simulink model "Ini_SO3_model_MixedCZ"  (R2021a)
settings: Solver=ode4  StartTime=0.0  StopTime=1000  FixedStep=0.02  RelTol=1e-3
values from neighbouring files (symbols this model uses):
  alpha = 0.05    [Ini_SO3.m]    (also in Ini_SO3_MixedCZ.m = 0.3; coneNew.m = acos(cosalpha))
  beta = 0.05    [Ini_SO3.m]    (also in Ini_SO3_MixedCZ.m = 0.3)
  G = [1,0,0 ... (first row only)    [Ini_SO3.m]    (also in Ini_SO3_MixedCZ.m; Symmetric test.m = inv(J)*D*E*D')
  J0 = [60 0 -5 ... (first row only)    [Ini_SO3.m]    (also in Ini_SO3_MixedCZ.m)
  J1 = [60 0 -5 ... (first row only)    [Ini_SO3.m]    (also in Ini_SO3_MixedCZ.m)
  J2 = [60 0 -5 ... (first row only)    [Ini_SO3.m]    (also in Ini_SO3_MixedCZ.m)
  J3 = [60 0 -5 ... (first row only)    [Ini_SO3.m]    (also in Ini_SO3_MixedCZ.m)
  K = [0.5,5,25,0.5]'    [Ini_SO3_MixedCZ.m]
  K1 = [0.01,0,30,0.2]'    [Ini_SO3.m]    (also in Ini_SO3_MixedCZ.m = [0.01,0,30,0.1]')
  lambda = 0.05    [Ini_SO3.m]    (also in Ini_SO3_MixedCZ.m = 0.3; SO3toThetan.m = diag(lambda))
  Omega01 = [0.03;0.02;-0.03]    [Ini_SO3.m]    (also in Ini_SO3_MixedCZ.m = [0,0,0])
  Omega02 = [-0.02;0.02;-0.03]    [Ini_SO3.m]    (also in Ini_SO3_MixedCZ.m = [0,0,0])
  Omega03 = [0;0.03;0.04]    [Ini_SO3.m]    (also in Ini_SO3_MixedCZ.m = [0,0,0])
  Omega0d = [0;0;0]    [Ini_SO3.m]    (also in Ini_SO3_MixedCZ.m)
  R01 = SO3(deg2rad(-80), nd0)    [Ini_SO3.m]    (also in Ini_SO3_MixedCZ.m = SO3(2.387, [0.3145,0.9113,0.2658]'))
  R02 = SO3(deg2rad(40),[0;1;1]/norm([0;1;1]))    [Ini_SO3.m]    (also in Ini_SO3_MixedCZ.m = SO3(1.422, [0.1772,0.9751,-0.1329]'))
  R03 = SO3(deg2rad(-120), nd0)    [Ini_SO3.m]    (also in Ini_SO3_MixedCZ.m = SO3(2.007, [0.2997,0.9415,0.1543]'))
  Rd = SO3(-(2*pi-Angd),nd)    [Ini_SO3.m]    (also in Ini_SO3_MixedCZ.m = SO3(Angd,nd))
  Rd0 = SO3(-(2*pi-Angd0),nd0)    [Ini_SO3.m]    (also in Ini_SO3_MixedCZ.m = SO3(Angd0,nd0))
  X = zeros(4,4)    [Ini_SO3.m]    (also in Ini_SO3_MixedCZ.m; coneNew.m = R .* cos(A))
undefined symbols (not defined in the file or in its folder): deg, rad, s
libraries: aerolibconvert2 x8
settings Model: Creator=Zeyu  LastModifiedBy=泽禹

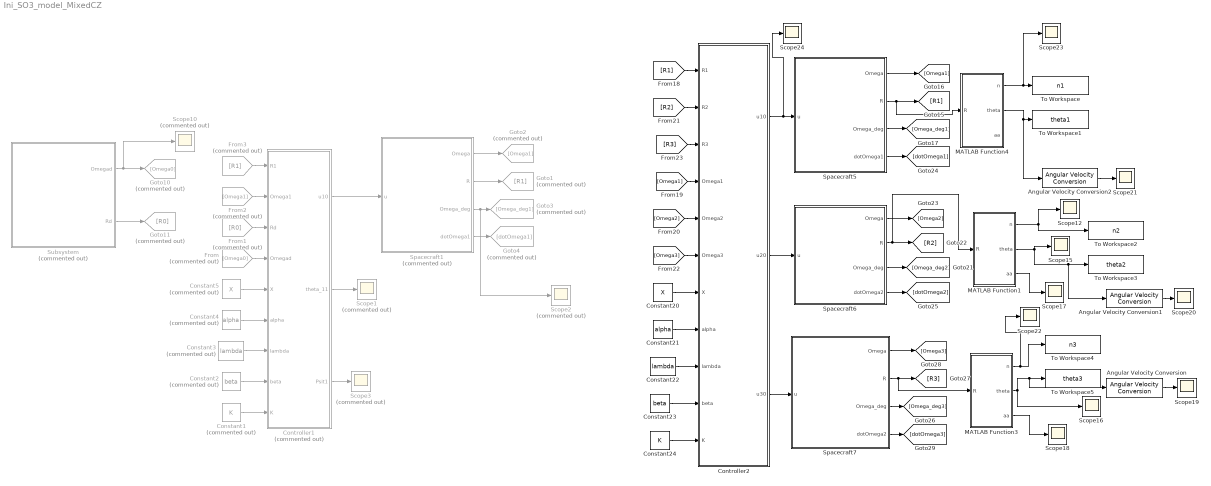
== system Ini_SO3_model_MixedCZ ==
  Angular Velocity Conversion : aerolibconvert2/Angular Velocity Conversion  IU=rad/s  OU=deg/s
  Angular Velocity Conversion1 : aerolibconvert2/Angular Velocity Conversion  IU=rad/s  OU=deg/s
  Angular Velocity Conversion2 : aerolibconvert2/Angular Velocity Conversion  IU=rad/s  OU=deg/s
  Constant1 : Constant  Commented=on  Value=K
  Constant2 : Constant  Commented=on  Value=beta
  Constant20 : Constant  Value=X
  Constant21 : Constant  Value=alpha
  Constant22 : Constant  Value=lambda
  Constant23 : Constant  Value=beta
  Constant24 : Constant  Value=K
  Constant3 : Constant  Commented=on  Value=lambda
  Constant4 : Constant  Commented=on  Value=alpha
  Constant5 : Constant  Commented=on  Value=X
  Controller1 : MATLAB Function  Commented=on  TreatAsAtomicUnit=on
  Controller2 : MATLAB Function  TreatAsAtomicUnit=on
  From : From  Commented=on  GotoTag=Omega0
  From1 : From  Commented=on  GotoTag=R0
  From2 : From  Commented=on  GotoTag=Omega1
  From3 : From  Commented=on  GotoTag=R1
  Goto1 : Goto  Commented=on  GotoTag=R1
  Goto10 : Goto  Commented=on  GotoTag=Omega0
  Goto11 : Goto  Commented=on  GotoTag=R0
  Goto2 : Goto  Commented=on  GotoTag=Omega1
  Goto3 : Goto  Commented=on  GotoTag=Omega_deg1
  Goto4 : Goto  Commented=on  GotoTag=dotOmega1
  MATLAB Function1 : MATLAB Function  TreatAsAtomicUnit=on
  MATLAB Function3 : MATLAB Function  TreatAsAtomicUnit=on
  MATLAB Function4 : MATLAB Function  TreatAsAtomicUnit=on
  Scope{1..3,10} (4 alike) : Scope  Commented=on
  Scope{12,15..24} (11 alike) : Scope
  Spacecraft1 : Subsystem  Commented=on
  Spacecraft5 : Subsystem
  Spacecraft6 : Subsystem
  Spacecraft7 : Subsystem
  Subsystem : Subsystem  Commented=on
  To Workspace : ToWorkspace  VariableName=n1  SampleTime=-1
  To Workspace1 : ToWorkspace  VariableName=theta1  SampleTime=-1
  To Workspace2 : ToWorkspace  VariableName=n2  SampleTime=-1
  To Workspace3 : ToWorkspace  VariableName=theta2  SampleTime=-1
  To Workspace4 : ToWorkspace  VariableName=n3  SampleTime=-1
  To Workspace5 : ToWorkspace  VariableName=theta3  SampleTime=-1
  wires:
  Spacecraft5/4(dotOmega1) -> [dotOmega1]
  Spacecraft5/3(Omega_deg) -> [Omega_deg1]
  Spacecraft6/3(Omega_deg) -> [Omega_deg2]
  Spacecraft6/1(Omega) -> [Omega2]
  Spacecraft6/4(dotOmega2) -> [dotOmega2]
  Spacecraft5/1(Omega) -> [Omega1]
  Spacecraft5/2(R) -> MATLAB Function4/1(R), [R1]
  Controller2/2(u20) -> Spacecraft6/1(u)
  Controller2/1(u10) -> Scope24/1, Spacecraft5/1(u)
  [R1] -> Controller2/1(R1)
  [Omega1] -> Controller2/4(Omega1)
  [Omega2] -> Controller2/5(Omega2)
  [R2] -> Controller2/2(R2)
  Constant20/1 -> Controller2/7(X)
  Constant21/1 -> Controller2/8(alpha)
  Constant22/1 -> Controller2/9(lambda)
  Constant23/1 -> Controller2/10(beta)
  Constant24/1 -> Controller2/11(K)
  Spacecraft7/3(Omega_deg) -> [Omega_deg3]
  Spacecraft7/4(dotOmega2) -> [dotOmega3]
  Controller2/3(u30) -> Spacecraft7/1(u)
  Spacecraft7/1(Omega) -> [Omega3]
  [Omega3] -> Controller2/6(Omega3)
  [R3] -> Controller2/3(R3)
  Spacecraft6/2(R) -> MATLAB Function1/1(R), [R2]
  Spacecraft7/2(R) -> MATLAB Function3/1(R), [R3]
  MATLAB Function4/1(n) -> Scope23/1, To Workspace/1
  MATLAB Function1/2(theta) -> Angular Velocity Conversion1/1, To Workspace3/1, Scope15/1
  MATLAB Function1/1(n) -> To Workspace2/1, Scope12/1
  MATLAB Function3/1(n) -> Scope22/1, To Workspace4/1
  MATLAB Function3/2(theta) -> Scope16/1, Angular Velocity Conversion/1, To Workspace5/1
  MATLAB Function1/3(aa) -> Scope17/1
  MATLAB Function3/3(aa) -> Scope18/1
  Angular Velocity Conversion/1 -> Scope19/1
  Angular Velocity Conversion1/1 -> Scope20/1
  Angular Velocity Conversion2/1 -> Scope21/1
  MATLAB Function4/2(theta) -> Angular Velocity Conversion2/1, To Workspace1/1
  Subsystem/2(Rd) -> Goto11/1
  Subsystem/1(Omegad) -> Scope10/1, Goto10/1
  Spacecraft1/2(R) -> Goto1/1
  Spacecraft1/3(Omega_deg) -> Scope2/1, Goto3/1
  Spacecraft1/1(Omega) -> Goto2/1
  Spacecraft1/4(dotOmega1) -> Goto4/1
  Controller1/1(u10) -> Spacecraft1/1(u)
  Constant1/1 -> Controller1/9(K)
  Controller1/2(theta_11) -> Scope1/1
  Constant2/1 -> Controller1/8(beta)
  Constant3/1 -> Controller1/7(lambda)
  Constant4/1 -> Controller1/6(alpha)
  Constant5/1 -> Controller1/5(X)
  From/1 -> Controller1/4(Omegad)
  From1/1 -> Controller1/3(Rd)
  From2/1 -> Controller1/2(Omega1)
  From3/1 -> Controller1/1(R1)
  Controller1/3(Psit1) -> Scope3/1

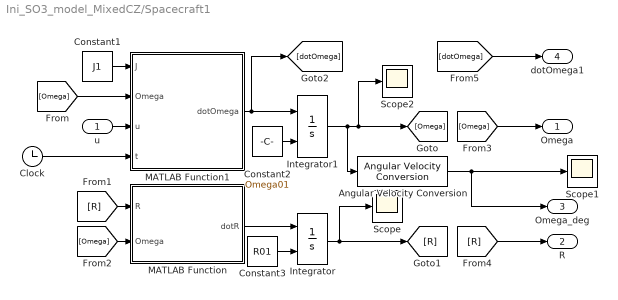
== system Ini_SO3_model_MixedCZ/Spacecraft1 ==
  u : Inport
  Angular Velocity Conversion : aerolibconvert2/Angular Velocity Conversion  IU=rad/s  OU=deg/s
  Clock : Clock
  Constant1 : Constant  Value=J1
  Constant2 : Constant  Value=Omega01
  Constant3 : Constant  Value=R01
  Integrator : Integrator  InitialConditionSource=external
  Integrator1 : Integrator  InitialConditionSource=external
  MATLAB Function : MATLAB Function  TreatAsAtomicUnit=on
  MATLAB Function1 : MATLAB Function  TreatAsAtomicUnit=on
  Scope : Scope
  Scope1 : Scope
  Scope2 : Scope
  Omega : Outport
  R : Outport  Port=2
  Omega_deg : Outport  Port=3
  dotOmega1 : Outport  Port=4
  wires:
  Constant3/1 -> Integrator/2
  Integrator/1 -> [R], Scope/1
  Constant1/1 -> MATLAB Function1/1(J)
  Integrator1/1 -> Scope2/1, [Omega], Angular Velocity Conversion/1
  MATLAB Function1/1(dotOmega) -> [dotOmega], Integrator1/1
  [Omega] -> MATLAB Function/2(Omega)
  MATLAB Function/1(dotR) -> Integrator/1
  Constant2/1 -> Integrator1/2
  [Omega] -> MATLAB Function1/2(Omega)
  [R] -> MATLAB Function/1(R)
  Angular Velocity Conversion/1 -> Omega_deg/1, Scope1/1
  u/1 -> MATLAB Function1/3(u)
  [Omega] -> Omega/1
  [R] -> R/1
  Clock/1 -> MATLAB Function1/4(t)
  [dotOmega] -> dotOmega1/1

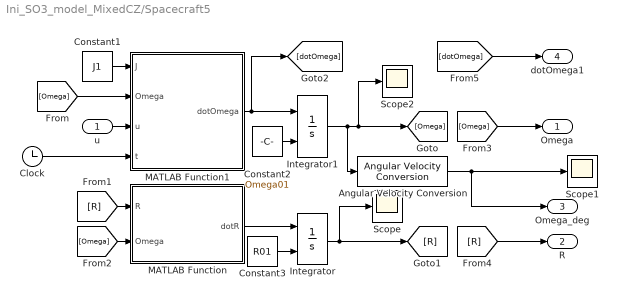
== system Ini_SO3_model_MixedCZ/Spacecraft5 ==
  u : Inport
  Angular Velocity Conversion : aerolibconvert2/Angular Velocity Conversion  IU=rad/s  OU=deg/s
  Clock : Clock
  Constant1 : Constant  Value=J1
  Constant2 : Constant  Value=Omega01
  Constant3 : Constant  Value=R01
  Integrator : Integrator  InitialConditionSource=external
  Integrator1 : Integrator  InitialConditionSource=external
  MATLAB Function : MATLAB Function  TreatAsAtomicUnit=on
  MATLAB Function1 : MATLAB Function  TreatAsAtomicUnit=on
  Scope : Scope
  Scope1 : Scope
  Scope2 : Scope
  Omega : Outport
  R : Outport  Port=2
  Omega_deg : Outport  Port=3
  dotOmega1 : Outport  Port=4
  wires:
  Constant3/1 -> Integrator/2
  Integrator/1 -> [R], Scope/1
  Constant1/1 -> MATLAB Function1/1(J)
  Integrator1/1 -> Scope2/1, [Omega], Angular Velocity Conversion/1
  MATLAB Function1/1(dotOmega) -> [dotOmega], Integrator1/1
  [Omega] -> MATLAB Function/2(Omega)
  MATLAB Function/1(dotR) -> Integrator/1
  Constant2/1 -> Integrator1/2
  [Omega] -> MATLAB Function1/2(Omega)
  [R] -> MATLAB Function/1(R)
  Angular Velocity Conversion/1 -> Omega_deg/1, Scope1/1
  u/1 -> MATLAB Function1/3(u)
  [Omega] -> Omega/1
  [R] -> R/1
  Clock/1 -> MATLAB Function1/4(t)
  [dotOmega] -> dotOmega1/1

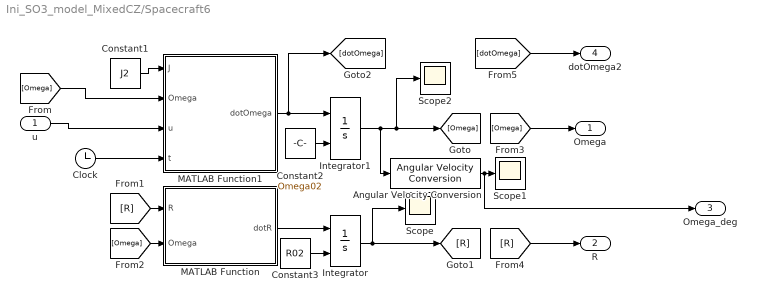
== system Ini_SO3_model_MixedCZ/Spacecraft6 ==
  u : Inport
  Angular Velocity Conversion : aerolibconvert2/Angular Velocity Conversion  IU=rad/s  OU=deg/s
  Clock : Clock
  Constant1 : Constant  Value=J2
  Constant2 : Constant  Value=Omega02
  Constant3 : Constant  Value=R02
  Integrator : Integrator  InitialConditionSource=external
  Integrator1 : Integrator  InitialConditionSource=external
  MATLAB Function : MATLAB Function  TreatAsAtomicUnit=on
  MATLAB Function1 : MATLAB Function  TreatAsAtomicUnit=on
  Scope : Scope
  Scope1 : Scope
  Scope2 : Scope
  Omega : Outport
  R : Outport  Port=2
  Omega_deg : Outport  Port=3
  dotOmega2 : Outport  Port=4
  wires:
  Constant3/1 -> Integrator/2
  Integrator/1 -> [R], Scope/1
  Constant1/1 -> MATLAB Function1/1(J)
  [Omega] -> MATLAB Function/2(Omega)
  MATLAB Function/1(dotR) -> Integrator/1
  Constant2/1 -> Integrator1/2
  [Omega] -> MATLAB Function1/2(Omega)
  [R] -> MATLAB Function/1(R)
  u/1 -> MATLAB Function1/3(u)
  [Omega] -> Omega/1
  [R] -> R/1
  Clock/1 -> MATLAB Function1/4(t)
  Angular Velocity Conversion/1 -> Omega_deg/1, Scope1/1
  Integrator1/1 -> Scope2/1, [Omega], Angular Velocity Conversion/1
  [dotOmega] -> dotOmega2/1
  MATLAB Function1/1(dotOmega) -> [dotOmega], Integrator1/1

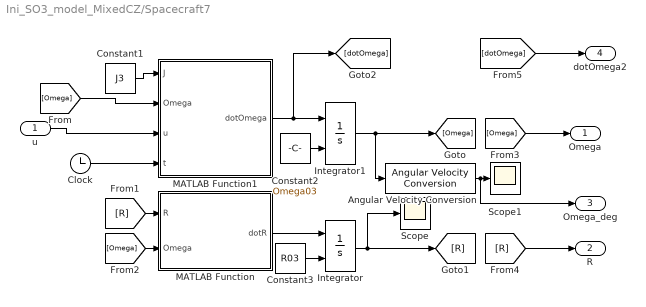
== system Ini_SO3_model_MixedCZ/Spacecraft7 ==
  u : Inport
  Angular Velocity Conversion : aerolibconvert2/Angular Velocity Conversion  IU=rad/s  OU=deg/s
  Clock : Clock
  Constant1 : Constant  Value=J3
  Constant2 : Constant  Value=Omega03
  Constant3 : Constant  Value=R03
  Integrator : Integrator  InitialConditionSource=external
  Integrator1 : Integrator  InitialConditionSource=external
  MATLAB Function : MATLAB Function  TreatAsAtomicUnit=on
  MATLAB Function1 : MATLAB Function  TreatAsAtomicUnit=on
  Scope : Scope
  Scope1 : Scope
  Omega : Outport
  R : Outport  Port=2
  Omega_deg : Outport  Port=3
  dotOmega2 : Outport  Port=4
  wires:
  Constant3/1 -> Integrator/2
  Integrator/1 -> [R], Scope/1
  Constant1/1 -> MATLAB Function1/1(J)
  Integrator1/1 -> [Omega], Angular Velocity Conversion/1
  [Omega] -> MATLAB Function/2(Omega)
  MATLAB Function/1(dotR) -> Integrator/1
  Constant2/1 -> Integrator1/2
  [Omega] -> MATLAB Function1/2(Omega)
  [R] -> MATLAB Function/1(R)
  u/1 -> MATLAB Function1/3(u)
  [Omega] -> Omega/1
  [R] -> R/1
  Clock/1 -> MATLAB Function1/4(t)
  Angular Velocity Conversion/1 -> Omega_deg/1, Scope1/1
  MATLAB Function1/1(dotOmega) -> [dotOmega], Integrator1/1
  [dotOmega] -> dotOmega2/1

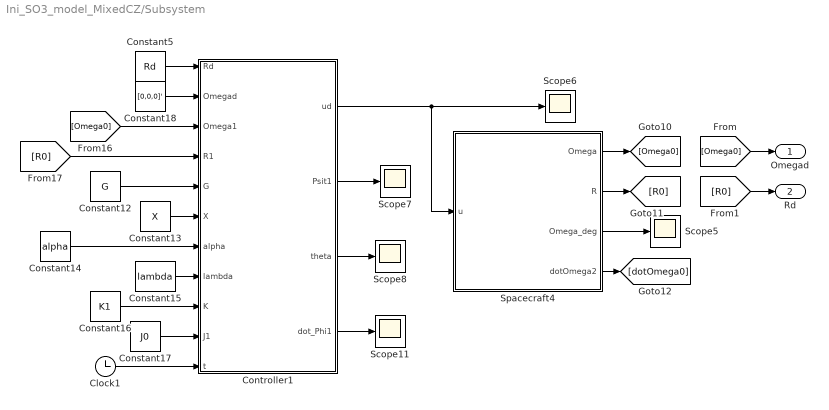
== system Ini_SO3_model_MixedCZ/Subsystem ==
  Clock1 : Clock
  Constant12 : Constant  Value=G
  Constant13 : Constant  Value=X
  Constant14 : Constant  Value=alpha
  Constant15 : Constant  Value=lambda
  Constant16 : Constant  Value=K1
  Constant17 : Constant  Value=J0
  Constant18 : Constant  Value=[0,0,0]'
  Constant5 : Constant  Value=Rd
  Controller1 : MATLAB Function  TreatAsAtomicUnit=on
  Scope{5..8,11} (5 alike) : Scope
  Spacecraft4 : Subsystem
  Omegad : Outport
  Rd : Outport  Port=2
  wires:
  Spacecraft4/4(dotOmega2) -> [dotOmega0]
  [R0] -> Controller1/4(R1)
  Controller1/1(ud) -> Scope6/1, Spacecraft4/1(u)
  Constant16/1 -> Controller1/9(K)
  Constant12/1 -> Controller1/5(G)
  Constant18/1 -> Controller1/2(Omegad)
  Constant17/1 -> Controller1/10(J1)
  Constant5/1 -> Controller1/1(Rd)
  Constant14/1 -> Controller1/7(alpha)
  Constant15/1 -> Controller1/8(lambda)
  Constant13/1 -> Controller1/6(X)
  Clock1/1 -> Controller1/11(t)
  [Omega0] -> Controller1/3(Omega1)
  Controller1/4(dot_Phi1) -> Scope11/1
  Controller1/3(theta) -> Scope8/1
  Spacecraft4/3(Omega_deg) -> Scope5/1
  Controller1/2(Psit1) -> Scope7/1
  Spacecraft4/2(R) -> [R0]
  Spacecraft4/1(Omega) -> [Omega0]
  [Omega0] -> Omegad/1
  [R0] -> Rd/1

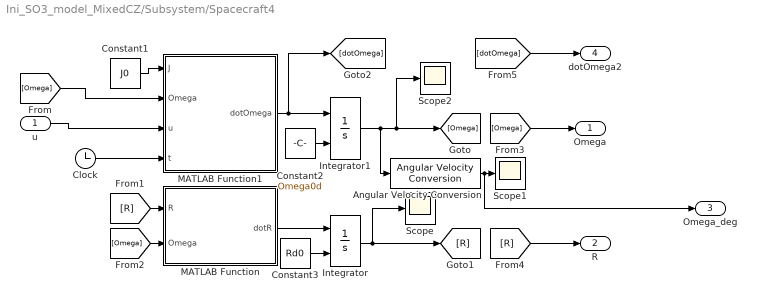
== system Ini_SO3_model_MixedCZ/Subsystem/Spacecraft4 ==
  u : Inport
  Angular Velocity Conversion : aerolibconvert2/Angular Velocity Conversion  IU=rad/s  OU=deg/s
  Clock : Clock
  Constant1 : Constant  Value=J0
  Constant2 : Constant  Value=Omega0d
  Constant3 : Constant  Value=Rd0
  Integrator : Integrator  InitialConditionSource=external
  Integrator1 : Integrator  InitialConditionSource=external
  MATLAB Function : MATLAB Function  TreatAsAtomicUnit=on
  MATLAB Function1 : MATLAB Function  TreatAsAtomicUnit=on
  Scope : Scope
  Scope1 : Scope
  Scope2 : Scope
  Omega : Outport
  R : Outport  Port=2
  Omega_deg : Outport  Port=3
  dotOmega2 : Outport  Port=4
  wires:
  MATLAB Function1/1(dotOmega) -> Integrator1/1, [dotOmega]
  [dotOmega] -> dotOmega2/1
  Integrator1/1 -> Angular Velocity Conversion/1, [Omega], Scope2/1
  Angular Velocity Conversion/1 -> Scope1/1, Omega_deg/1
  Clock/1 -> MATLAB Function1/4(t)
  [R] -> R/1
  [Omega] -> Omega/1
  u/1 -> MATLAB Function1/3(u)
  [R] -> MATLAB Function/1(R)
  [Omega] -> MATLAB Function1/2(Omega)
  Constant2/1 -> Integrator1/2
  MATLAB Function/1(dotR) -> Integrator/1
  [Omega] -> MATLAB Function/2(Omega)
  Constant1/1 -> MATLAB Function1/1(J)
  Integrator/1 -> Scope/1, [R]
  Constant3/1 -> Integrator/2

== matlab function Ini_SO3_model_MixedCZ/Controller1 ==
  settings: updateMethod=DISCRETE
  data: R1 input; Omega1 input; Rd input; Omegad input; u10 output; X input; alpha input; lambda input; beta input; K input; theta_11 output; Psit1 output
function [u10,theta_11,Psit1]   = fcn(R1,Omega1,Rd,Omegad,X,alpha,lambda,beta,K)
% X = n*4, 4= 1*3+1;
   u10=zeros(3,1);
G = [1,0,0;
     0,1,0;
     0,0,1];

    %% Mixed attitude constraints
    tel = [0.750,0.433,0.500]'; %telescope
    ant = [0,1,0]'; %antenna
    tru= [-1,0,0;0,-1,0;0,0,-1]';  %three trust
 
        
    Phi1 = 1;
    P_Phi1 = zeros(3,1);
    
    Psit1 =0.5*trace(G*(eye(3)-Rd'*R1));
    e_R1t = x_hat2x(G*Rd'*R1-R1'*Rd*G);
    e_omega_t_1=Omega1-R1'*Rd*Omegad;
    
    n=(size(X,1));
    theta_11=zeros(4,1);
for i = 1:n
    if i<n % static attitude-forbidden zones
        Phi1 = Phi1  + (-alpha * log((cos(X(i,end))-tel'*R1'*X(i,1:3)')/(1+cos(X(i,end)))));
        P_Phi1 = P_Phi1 ...
            + (alpha*(x2x_hat(R1'*X(i,1:3)')*tel)/(tel'*R1'*X(i,1:3)'-cos(X(i,end))));
       theta_11(i)=rad2deg(acos(tel'*R1'*X(i,1:3)')); 
    end
    if i==n % the attitude-mandatory zones
        Phi1 = Phi1  + (-lambda * log((ant'*R1'*X(i,1:3)'-cos(X(i,end)))/(1+cos(X(i,end)))));
        P_Phi1 = P_Phi1 ...
            + (lambda*(x2x_hat(R1'*X(i,1:3)')*ant)/(ant'*R1'*X(i,1:3)'-cos(X(i,end))));
        theta_11(i)=rad2deg(acos(ant'*R1'*X(i,1:3)'));
    end
end

% if flag==0 
%% 传统不考虑饱和控制器 
ksi=0.001;
S1=Omega1/((norm(Omega1))^2+ksi);
F1=e_R1t*Phi1+Psit1*P_Phi1;

u10=-K(2)*e_R1t-K(3)*(e_omega_t_1)-K(4)*F1;
end

== matlab function Ini_SO3_model_MixedCZ/Subsystem/Spacecraft4/MATLAB Function ==
  data: R input; dotR output; Omega input
function dotR  = fcn(R, Omega)
    Omega_x = [0 -Omega(3) Omega(2);
              Omega(3) 0  -Omega(1);
              -Omega(2) Omega(1) 0];
%           [x1,y1]=eig(R);
%           
%           n=real(x1(:,3));
%           a=R*n-n;
%           theta = acos((trace(R)-1)/2);

    dotR = R*Omega_x;

== matlab function Ini_SO3_model_MixedCZ/Subsystem/Spacecraft4/MATLAB Function1 ==
  data: J input; dotOmega output; Omega input; u input; t input
function dotOmega = fcn(J, Omega, u, t)
    Omega_x = [0 -Omega(3) Omega(2);
              Omega(3) 0  -Omega(1);
              -Omega(2) Omega(1) 0];
    d=10^-3*[-1+3*sin(0.1*t+pi/2)+4*sin(0.003*t);
    1.5-1.5*sin(0.02*t)-3*sin(0.05*t+pi/2);
    1+2*sin(0.1*t)-1.5*sin(0.04*t+pi/2)];

%     dotOmega = J\(u-Omega_x*J*Omega+d);
    dotOmega = J\(u-Omega_x*J*Omega);

== matlab function Ini_SO3_model_MixedCZ/Subsystem/Controller1 ==
  settings: updateMethod=DISCRETE
  data: Rd input; Omegad input; Omega1 input; R1 input; G input; ud output; X input; alpha input; lambda input; K input; J1 input; Psit1 output; theta output; t input; dot_Phi1 output
function [ud,Psit1,theta,dot_Phi1]  = fcn(Rd,Omegad,Omega1,R1,G,X,alpha,lambda,K,J1,t)
% X = n*4, 4= 1*3+1;
ud=zeros(3,1);
    %% Attitude Error Function
    
    Psit1 =0.5*trace(G*(eye(3)-Rd'*R1));
    
    e_R1t = x_hat2x(G*Rd'*R1-R1'*Rd*G);
    
    e_omega_1=Omega1-R1'*Rd*Omegad;
    
    
    %% Attitude Error Dynamics

%     dot_Psit1 = e_omega_1'*e_R1t;
    dot_Psit1 = e_R1t;
    
    %% Mixed attitude constraints
    tel = [0.750,0.433,0.500]'; %telescope
    ant = [0,1,0]'; %antenna
    
    aa=R1*ant;
    
    Phi1 = 1;
    dot_Phi1 = zeros(3,1);
    n=(size(X,1));
    theta=zeros(4,1);
%     Ang=deg2rad(10);
%     flag=zeros(4,1);
% for i = 1:n
%     theta(i)=rad2deg(acos(tel'*R1'*X(i,1:3)'));
%     if i<n % static attitude-forbidden zones
%          if (cos(X(i,end)+Ang)-tel'*R1'*X(i,1:3)')<=0
%             Phi1=Phi1+alpha*(tel'*R1'*X(i,1:3)'-cos(X(i,end)+Ang))^2/2;
%             dot_Phi1 = dot_Phi1-alpha*(tel'*R1'*X(i,1:3)'-cos(X(i,end)+Ang))*(x2x_hat(R1'*X(i,1:3)')*tel);
%             if(cos(X(i,end))-tel'*R1'*X(i,1:3)')<=0
%                 flag(i)=1;
%             end
%          end 
%     end
%      if i==n % the attitude-mandatory zones
%          theta(i)=rad2deg(acos(ant'*R1'*X(i,1:3)'));
%          if (cos(X(i,end)-Ang)-ant'*R1'*X(i,1:3)')>=0
%             Phi1 = Phi1 + lambda*(cos(X(i,end)-Ang)-ant'*R1'*X(i,1:3)')^2/2;
%             dot_Phi1 = dot_Phi1+lambda *(cos(X(i,end)-Ang)-ant'*R1'*X(i,1:3)')*(x2x_hat(R1'*X(i,1:3)')*ant);
%             if (cos(X(i,end))-ant'*R1'*X(i,1:3)')>=0
%                 flag(i)=1;
%             end
%          end
%     end
% end

% if flag==0 
%% 传统不考虑饱和控制器 
        for i = 1:n
                if i<n % static attitude-forbidden zones
                         Phi1 = Phi1  + (-alpha * log((cos(X(i,end))-tel'*R1'*X(i,1:3)')/(1+cos(X(i,end)))));
                        dot_Phi1 = dot_Phi1 ...
                        + (alpha*(x2x_hat(R1'*X(i,1:3)')*tel)/(tel'*R1'*X(i,1:3)'-cos(X(i,end))));
                    theta(i)=rad2deg(acos(tel'*R1'*X(i,1:3)'));
                end
                 if i==n % the attitude-mandatory zones
                    theta(i)=rad2deg(acos(ant'*R1'*X(i,1:3)'));
                        Phi1 = Phi1  + (-lambda * log((ant'*R1'*X(i,1:3)'-cos(X(i,end)))/(1+cos(X(i,end)))));
                        dot_Phi1 = dot_Phi1 ...
                            + (lambda*(x2x_hat(R1'*X(i,1:3)')*ant)/(ant'*R1'*X(i,1:3)'-cos(X(i,end))));
                 end
        end
%      if t>=30
        ksi=0.001; % 滑模平滑项
        S1=Omega1/((norm(Omega1)^2)+ksi);
        ud=-K(1)*Psit1*S1-K(3)*Omega1-K(4)*(Psit1*dot_Phi1+e_R1t*Phi1);
%      else
%         ud=[0,0,0]';
%      end
%     else 
%         gamma1=0.8;
%         Omega1_gamma=[sign(Omega1(1))*abs(Omega1(1))^gamma1;sign(Omega1(2))*abs(Omega1(2))^gamma1;sign(Omega1(3))*abs(Omega1(3))^gamma1];
%         ud=-K(3)*Omega1-0.1*K(3)*Omega1_gamma-K(2)*dot_Phi1-K(2)*0.01*Phi1*(Omega1)/(norm(Omega1)+0.001)-K(2)*0.01*Phi1*(Omega1)/(norm(Omega1)+0.001);
%     end

% S1=e_omega_1/((norm(e_omega_1)^2)+ksi);
% dotVR1=dot_Psit1*Phi1+Psit1*dot_Phi1;

% ud=-K(2)/gamma1*e_R1t-K(3)/gamma1*e_omega_1...
%     -K(4)/gamma1*dotVR1; %no disturbence
% ud=-K(2)/gamma1*e_R1t-K(3)/gamma1*e_omega_1...
%    +x2x_hat(Omega1)*J1*Omega1; %no disturbence
end

== matlab function Ini_SO3_model_MixedCZ/Spacecraft5/MATLAB Function ==
  data: R input; dotR output; Omega input
function dotR  = fcn(R, Omega)
    Omega_x = [0 -Omega(3) Omega(2);
              Omega(3) 0  -Omega(1);
              -Omega(2) Omega(1) 0];
%           [x1,y1]=eig(R);
%           
%           n=real(x1(:,3));
%           a=R*n-n;
%           theta = acos((trace(R)-1)/2);

    dotR = R*Omega_x;

== matlab function Ini_SO3_model_MixedCZ/Spacecraft5/MATLAB Function1 ==
  data: J input; dotOmega output; Omega input; u input; t input
function dotOmega = fcn(J, Omega, u, t)
    Omega_x = [0 -Omega(3) Omega(2);
              Omega(3) 0  -Omega(1);
              -Omega(2) Omega(1) 0];
    d=10^-3*[-1+3*sin(0.1*t+pi/2)+4*sin(0.003*t);
    1.5-1.5*sin(0.02*t)-3*sin(0.05*t+pi/2);
    1+2*sin(0.1*t)-1.5*sin(0.04*t+pi/2)];
   dotOmega=zeros(3,1);
%     dotOmega = J\(u-Omega_x*J*Omega+d);
    dotOmega = J\(u-Omega_x*J*Omega);

== matlab function Ini_SO3_model_MixedCZ/Spacecraft6/MATLAB Function ==
  data: R input; dotR output; Omega input
function dotR  = fcn(R, Omega)
    Omega_x = [0 -Omega(3) Omega(2);
              Omega(3) 0  -Omega(1);
              -Omega(2) Omega(1) 0];
%           [x1,y1]=eig(R);
%           
%           n=real(x1(:,3));
%           a=R*n-n;
%           theta = acos((trace(R)-1)/2);

    dotR = R*Omega_x;

== matlab function Ini_SO3_model_MixedCZ/Spacecraft6/MATLAB Function1 ==
  data: J input; dotOmega output; Omega input; u input; t input
function dotOmega = fcn(J, Omega, u, t)
    Omega_x = [0 -Omega(3) Omega(2);
              Omega(3) 0  -Omega(1);
              -Omega(2) Omega(1) 0];
    d=10^-3*[-1+3*sin(0.1*t+pi/2)+4*sin(0.003*t);
    1.5-1.5*sin(0.02*t)-3*sin(0.05*t+pi/2);
    1+2*sin(0.1*t)-1.5*sin(0.04*t+pi/2)];
    dotOmega=zeros(3,1);
%     dotOmega = J\(u-Omega_x*J*Omega+d);
    dotOmega = J\(u-Omega_x*J*Omega);

== matlab function Ini_SO3_model_MixedCZ/Controller2 ==
  settings: updateMethod=DISCRETE
  data: R1 input; R2 input; R3 input; Omega1 input; Omega2 input; Omega3 input; u10 output; u20 output; u30 output; X input; alpha input; lambda input; beta input; K input
function [u10,u20,u30]  = fcn(R1,R2,R3,Omega1,Omega2,Omega3,X,alpha,lambda,beta,K)
% X = n*4, 4= 1*3+1;
u10=zeros(3,1);
u20=zeros(3,1);
u30=zeros(3,1);
    %% Mixed attitude constraints
    tel = [0.750,0.433,0.500]'; %telescope
    ant = [0,1,0]'; %antenna
    tru= [-1,0,0;0,-1,0;0,0,-1]';  %three trust
    
        
    Phi1 = 1;
    dot_Phi1 = zeros(3,1);
    
    Phi2 = 1;
    dot_Phi2 = zeros(3,1);
    
    Phi3 = 1;
    dot_Phi3 = zeros(3,1);
    
    n=(size(X,1));

    Ang1=deg2rad(20);
    Ang2=deg2rad(10);
    Ang3=deg2rad(5);
    thate_T=deg2rad(15);
    
for i = 1:n+1
%     theta1(i)=rad2deg(acos(tel'*R1'*X(i,1:3)'));
    if i<n % static attitude-forbidden zones
%         theta1(i)=rad2deg(acos(tel'*R1'*X(i,1:3)'));
%         theta2(i)=rad2deg(acos(tel'*R2'*X(i,1:3)'));
         if (cos(X(i,end)+Ang1)-tel'*R1'*X(i,1:3)')<=0
            Phi1=Phi1+alpha*(tel'*R1'*X(i,1:3)'-cos(X(i,end)+Ang1))^2/2;
            dot_Phi1 = dot_Phi1-alpha*(tel'*R1'*X(i,1:3)'-cos(X(i,end)+Ang1))*(x2x_hat(R1'*X(i,1:3)')*tel);
         end
%          if (cos(X(i,end))-tel'*R1'*X(i,1:3)')<=0
%              flag1(i)=1;
%          end
         if (cos(X(i,end)+Ang1)-tel'*R2'*X(i,1:3)')<=0
            Phi2=Phi2+alpha*(tel'*R2'*X(i,1:3)'-cos(X(i,end)+Ang1))^2/2;
            dot_Phi2 = dot_Phi2-alpha*(tel'*R2'*X(i,1:3)'-cos(X(i,end)+Ang1))*(x2x_hat(R2'*X(i,1:3)')*tel);
         end
%          if (cos(X(i,end))-tel'*R2'*X(i,1:3)')<=0
%              flag2(i)=0;
%          end
         if (cos(X(i,end)+Ang1)-tel'*R3'*X(i,1:3)')<=0
            Phi3=Phi3+alpha*(tel'*R3'*X(i,1:3)'-cos(X(i,end)+Ang1))^2/2;
            dot_Phi3 = dot_Phi3-alpha*(tel'*R3'*X(i,1:3)'-cos(X(i,end)+Ang1))*(x2x_hat(R3'*X(i,1:3)')*tel);
         end
    end
     if i==n % the attitude-mandatory zones
%          theta1(i)=rad2deg(acos(ant'*R1'*X(i,1:3)'));
%         theta1(i)=rad2deg(acos(ant'*R1'*X(i,1:3)'));
%         theta2(i)=rad2deg(acos(ant'*R2'*X(i,1:3)'));
         if (cos(X(i,end)-Ang2)-ant'*R1'*X(i,1:3)')>=0
            Phi1 = Phi1 + lambda*(cos(X(i,end)-Ang2)-ant'*R1'*X(i,1:3)')^2/2;
            dot_Phi1 = dot_Phi1+lambda *(cos(X(i,end)-Ang2)-ant'*R1'*X(i,1:3)')*(x2x_hat(R1'*X(i,1:3)')*ant);
         end
%          if (cos(X(i,end))-ant'*R1'*X(i,1:3)')>=0
%              flag1(i)=1;
%          end
         if (cos(X(i,end)-Ang2)-ant'*R2'*X(i,1:3)')>=0
            Phi2 = Phi2 + lambda*(cos(X(i,end)-Ang2)-ant'*R2'*X(i,1:3)')^2/2;
            dot_Phi2 = dot_Phi2+lambda *(cos(X(i,end)-Ang2)-ant'*R2'*X(i,1:3)')*(x2x_hat(R2'*X(i,1:3)')*ant);
         end
%          if (cos(X(i,end))-ant'*R2'*X(i,1:3)')>=0
%              flag2(i)=1;
%          end

         if (cos(X(i,end)-Ang2)-ant'*R3'*X(i,1:3)')>=0
            Phi3 = Phi3 + lambda*(cos(X(i,end)-Ang2)-ant'*R3'*X(i,1:3)')^2/2;
            dot_Phi3 = dot_Phi3+lambda *(cos(X(i,end)-Ang2)-ant'*R3'*X(i,1:3)')*(x2x_hat(R3'*X(i,1:3)')*ant);
         end
     end
    if i==n+1
        for j=1:3  % three trust
%            theta12(j)=rad2deg(acos(tel'*R1'*R2*tru(j,:)'));
%            theta21(j)=rad2deg(acos(tel'*R2'*R1*tru(j,:)'));
%          theta2(i)=rad2deg(acos(ant'*R1'*X(i,1:3)'));
            if (cos(thate_T+Ang3)-tel'*R1'*R2*tru(j,:)')<=0
                Phi1=Phi1+beta*(tel'*R1'*R2*tru(j,:)'-cos(thate_T+Ang3))^2/2;
                dot_Phi1 = dot_Phi1-beta*(tel'*R1'*R2*tru(j,:)'-cos(thate_T+Ang3))*(x2x_hat(R1'*R2*tru(j,:)')*tel);
            end
            if (cos(thate_T+Ang3)-tel'*R1'*R3*tru(j,:)')<=0
                Phi1=Phi1+beta*(tel'*R1'*R3*tru(j,:)'-cos(thate_T+Ang3))^2/2;
                dot_Phi1 = dot_Phi1-beta*(tel'*R1'*R3*tru(j,:)'-cos(thate_T+Ang3))*(x2x_hat(R1'*R3*tru(j,:)')*tel);
            end
%             if (cos(thate_T)-tel'*R1'*R2*tru(j,:)')<=0
%              flag12(j)=1;
%             end
            if (cos(thate_T+Ang3)-tel'*R2'*R1*tru(j,:)')<=0
                Phi2=Phi2+beta*(tel'*R2'*R1*tru(j,:)'-cos(thate_T+Ang3))^2/2;
                dot_Phi2 = dot_Phi2-beta*(tel'*R2'*R1*tru(j,:)'-cos(thate_T+Ang3))*(x2x_hat(R2'*R1*tru(j,:)')*tel);
            end
            if (cos(thate_T+Ang3)-tel'*R2'*R3*tru(j,:)')<=0
                Phi2=Phi2+beta*(tel'*R2'*R3*tru(j,:)'-cos(thate_T+Ang3))^2/2;
                dot_Phi2 = dot_Phi2-beta*(tel'*R2'*R3*tru(j,:)'-cos(thate_T+Ang3))*(x2x_hat(R2'*R3*tru(j,:)')*tel);
            end
%             if (cos(thate_T)-tel'*R2'*R1*tru(j,:)')<=0
%              flag21(j)=1;
%             end
            if (cos(thate_T+Ang3)-tel'*R3'*R1*tru(j,:)')<=0
                Phi3=Phi3+beta*(tel'*R3'*R1*tru(j,:)'-cos(thate_T+Ang3))^2/2;
                dot_Phi3 = dot_Phi3-beta*(tel'*R3'*R1*tru(j,:)'-cos(thate_T+Ang3))*(x2x_hat(R3'*R1*tru(j,:)')*tel);
            end
            if (cos(thate_T+Ang3)-tel'*R3'*R2*tru(j,:)')<=0
                Phi3=Phi3+beta*(tel'*R3'*R2*tru(j,:)'-cos(thate_T+Ang3))^2/2;
                dot_Phi3 = dot_Phi3-beta*(tel'*R3'*R2*tru(j,:)'-cos(thate_T+Ang3))*(x2x_hat(R3'*R2*tru(j,:)')*tel);
            end
        end
    end

% if flag==0 
%% 传统不考虑饱和控制器 
  
        gamma1=0.8;
        Omega1_gamma=[sign(Omega1(1))*abs(Omega1(1))^gamma1;sign(Omega1(2))*abs(Omega1(2))^gamma1;sign(Omega1(3))*abs(Omega1(3))^gamma1];
        Omega2_gamma=[sign(Omega2(1))*abs(Omega2(1))^gamma1;sign(Omega2(2))*abs(Omega2(2))^gamma1;sign(Omega2(3))*abs(Omega2(3))^gamma1];
        Omega3_gamma=[sign(Omega2(1))*abs(Omega2(1))^gamma1;sign(Omega2(2))*abs(Omega2(2))^gamma1;sign(Omega2(3))*abs(Omega2(3))^gamma1];
        u10=-K(3)*Omega1-0.1*K(3)*Omega1_gamma-K(2)*dot_Phi1-K(2)*0.01*Phi1*(Omega1)/(norm(Omega1)+0.001)-K(2)*0.01*Phi1*(Omega1)/(norm(Omega1)+0.001);
        u20=-K(3)*Omega2-0.1*K(3)*Omega2_gamma-K(2)*dot_Phi2-K(2)*0.01*Phi2*(Omega2)/(norm(Omega2)+0.001)-K(2)*0.01*Phi2*(Omega2)/(norm(Omega2)+0.001);
        u30=-K(3)*Omega3-0.1*K(3)*Omega3_gamma-K(2)*dot_Phi3-K(2)*0.01*Phi3*(Omega3)/(norm(Omega3)+0.001)-K(2)*0.01*Phi3*(Omega3)/(norm(Omega3)+0.001);
end

% S1=e_omega_1/((norm(e_omega_1)^2)+ksi);
% dotVR1=dot_Psit1*Phi1+Psit1*dot_Phi1;

% ud=-K(2)/gamma1*e_R1t-K(3)/gamma1*e_omega_1...
%     -K(4)/gamma1*dotVR1; %no disturbence
% ud=-K(2)/gamma1*e_R1t-K(3)/gamma1*e_omega_1...
%    +x2x_hat(Omega1)*J1*Omega1; %no disturbence
end

== matlab function Ini_SO3_model_MixedCZ/MATLAB Function4 ==
  data: R input; n output; theta output; aa output
function [n,theta,aa]   = fcn(R)
    %So3 到轴角
    n=zeros(3,1);
    theta=0;
    
    n=zeros(3,1);
    theta=0;
    aa=0;
    theta=acos((trace(R)-1)/2);
    [A,lambda]=eig(R);
    lambda=real(lambda);
    lambda=diag(lambda);
    a=1;
    for i=1:3
        if lambda(i)>=0.99
            a=i;
            aa=1;
        end
    end
    b=a;
    n_temp=A(:,b);
    n_temp=n_temp/norm(n_temp);
    n1=real(n_temp(1));
    n2=real(n_temp(2));
    n3=real(n_temp(3));
   n=[n1;n2;n3];
end

== matlab function Ini_SO3_model_MixedCZ/Spacecraft7/MATLAB Function ==
  data: R input; dotR output; Omega input
function dotR  = fcn(R, Omega)
    Omega_x = [0 -Omega(3) Omega(2);
              Omega(3) 0  -Omega(1);
              -Omega(2) Omega(1) 0];
%           [x1,y1]=eig(R);
%           
%           n=real(x1(:,3));
%           a=R*n-n;
%           theta = acos((trace(R)-1)/2);

    dotR = R*Omega_x;

== matlab function Ini_SO3_model_MixedCZ/Spacecraft7/MATLAB Function1 ==
  data: J input; dotOmega output; Omega input; u input; t input
function dotOmega = fcn(J, Omega, u, t)
    Omega_x = [0 -Omega(3) Omega(2);
              Omega(3) 0  -Omega(1);
              -Omega(2) Omega(1) 0];
    d=10^-3*[-1+3*sin(0.1*t+pi/2)+4*sin(0.003*t);
    1.5-1.5*sin(0.02*t)-3*sin(0.05*t+pi/2);
    1+2*sin(0.1*t)-1.5*sin(0.04*t+pi/2)];
    dotOmega=zeros(3,1);
%     dotOmega = J\(u-Omega_x*J*Omega+d);
    dotOmega = J\(u-Omega_x*J*Omega);

== matlab function Ini_SO3_model_MixedCZ/MATLAB Function1 ==
  data: R input; n output; theta output; aa output
function [n,theta,aa]   = fcn(R)
    %So3 到轴角
    n=zeros(3,1);
    theta=0;
    
    n=zeros(3,1);
    theta=0;
    aa=0;
    theta=acos((trace(R)-1)/2);
    [A,lambda]=eig(R);
    lambda=real(lambda);
    lambda=diag(lambda);
    a=1;
    for i=1:3
        if lambda(i)>=0.99
            a=i;
            aa=1;
        end
    end
    b=a;
    n_temp=A(:,b);
    n_temp=n_temp/norm(n_temp);
    n1=real(n_temp(1));
    n2=real(n_temp(2));
    n3=real(n_temp(3));
   n=[n1;n2;n3];
end

== matlab function Ini_SO3_model_MixedCZ/MATLAB Function3 ==
  data: R input; n output; theta output; aa output
function [n,theta,aa]   = fcn(R)
    %So3 到轴角
    n=zeros(3,1);
    theta=0;
    
    n=zeros(3,1);
    theta=0;
    aa=0;
    theta=acos((trace(R)-1)/2);
    [A,lambda]=eig(R);
    lambda=real(lambda);
    lambda=diag(lambda);
    a=1;
    for i=1:3
        if lambda(i)>=0.99
            a=i;
            aa=1;
        end
    end
    b=a;
    n_temp=A(:,b);
    n_temp=n_temp/norm(n_temp);
    n1=real(n_temp(1));
    n2=real(n_temp(2));
    n3=real(n_temp(3));
   n=[n1;n2;n3];
end

== matlab function Ini_SO3_model_MixedCZ/Spacecraft1/MATLAB Function ==
  data: R input; dotR output; Omega input
function dotR  = fcn(R, Omega)
    Omega_x = [0 -Omega(3) Omega(2);
              Omega(3) 0  -Omega(1);
              -Omega(2) Omega(1) 0];
%           [x1,y1]=eig(R);
%           
%           n=real(x1(:,3));
%           a=R*n-n;
%           theta = acos((trace(R)-1)/2);

    dotR = R*Omega_x;

== matlab function Ini_SO3_model_MixedCZ/Spacecraft1/MATLAB Function1 ==
  data: J input; dotOmega output; Omega input; u input; t input
function dotOmega = fcn(J, Omega, u, t)
    Omega_x = [0 -Omega(3) Omega(2);
              Omega(3) 0  -Omega(1);
              -Omega(2) Omega(1) 0];
    d=10^-3*[-1+3*sin(0.1*t+pi/2)+4*sin(0.003*t);
    1.5-1.5*sin(0.02*t)-3*sin(0.05*t+pi/2);
    1+2*sin(0.1*t)-1.5*sin(0.04*t+pi/2)];
   dotOmega=zeros(3,1);
%     dotOmega = J\(u-Omega_x*J*Omega+d);
    dotOmega = J\(u-Omega_x*J*Omega);
